simulink model "sampleModel2_EMI_Var"  (R2017a)
settings: Solver=VariableStepAuto  StartTime=0.0  StopTime=10.0  RelTol=1e-3
undefined symbols (not defined in the file or in its folder): DiscIntNeverNeededParam
libraries: simulink x42
settings Model: Creator=cyfuzz  LastModifiedBy=cyfuzz

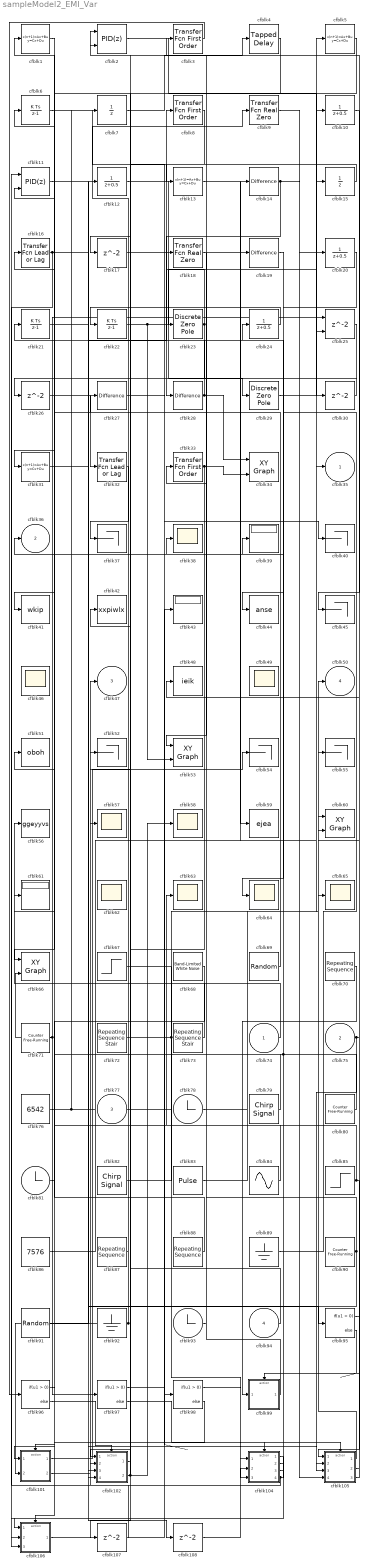
== system sampleModel2_EMI_Var ==
  cfblk74 : Inport
  cfblk75 : Inport  Port=2
  cfblk77 : Inport  Port=3
  cfblk94 : Inport  Port=4
  cfblk{1,5,13,31} (4 alike) : DiscreteStateSpace
  cfblk{10,12,20,24} (4 alike) : DiscreteTransferFcn  SampleTime=1
  cfblk101 : Subsystem  TreatAsAtomicUnit=on
  cfblk102 : Subsystem  TreatAsAtomicUnit=on
  cfblk104 : Subsystem  TreatAsAtomicUnit=on
  cfblk105 : Subsystem  TreatAsAtomicUnit=on
  cfblk106 : Subsystem  TreatAsAtomicUnit=on
  cfblk{17,26,30,107..108} (5 alike) : Delay  SampleTime=1
  cfblk11 : simulink/Continuous/PID Controller (2DOF)  Controller=PID  TimeDomain=Discrete-time  SampleTime=1  IntegratorMethod=Forward Euler  FilterMethod=Forward Euler  Form=Parallel  UseFilter=on  ControllerParametersSource=internal  P=1  I=1  D=0  N=100  b=1  c=1  InitialConditionSource=internal  InitialConditionForIntegrator=0  InitialConditionForFilter=0  ExternalReset=none  LimitOutput=off  UpperSaturationLimit=inf  LowerSaturationLimit=-inf  LinearizeAsGain=off  AntiWindupMode=none  Kb=1  TrackingMode=off  Kt=1  PParamMin=[]  PParamMax=[]  IParamMin=[]  IParamMax=[]  DParamMin=[]  DParamMax=[]  NParamMin=[]  NParamMax=[]  bParamMin=[]  bParamMax=[]  cParamMin=[]  cParamMax=[]  KbParamMin=[]  KbParamMax=[]  KtParamMin=[]  KtParamMax=[]  POutMin=[]  POutMax=[]  IOutMin=[]  IOutMax=[]  DOutMin=[]  DOutMax=[]  NOutMin=[]  NOutMax=[]  bOutMin=[]  bOutMax=[]  cOutMin=[]  cOutMax=[]  KbOutMin=[]  KbOutMax=[]  KtOutMin=[]  KtOutMax=[]  IntegratorOutMin=[]  IntegratorOutMax=[]  FilterOutMin=[]  FilterOutMax=[]  SumOutMin=[]  SumOutMax=[]  Sum1OutMin=[]  Sum1OutMax=[]  Sum2OutMin=[]  Sum2OutMax=[]  Sum3OutMin=[]  Sum3OutMax=[]  SumI1OutMin=[]  SumI1OutMax=[]  SumI2OutMin=[]  SumI2OutMax=[]  SumI3OutMin=[]  SumI3OutMax=[]  SumDOutMin=[]  SumDOutMax=[]  SaturationOutMin=[]  SaturationOutMax=[]  IntegratorContinuousStateAttributes=''  IntegratorStateMustResolveToSignalObject=off  IntegratorRTWStateStorageClass=Auto  FilterContinuousStateAttributes=''  FilterStateMustResolveToSignalObject=off  FilterRTWStateStorageClass=Auto  DifferentiatorICPrevScaledInput=0  DifferentiatorOutMin=[]  DifferentiatorOutMax=[]  InitialConditionSetting=State (most efficient)
  cfblk{14,19,27..28} (4 alike) : simulink/Discrete/Difference  ICPrevInput=0.0  OutMin=[]  OutMax=[]  OutDataTypeStr=Inherit: Inherit via back propagation  OutDataType=fixdt(1, 16)  OutScaling=2^-10  DoSatur=off
  cfblk15 : UnitDelay
  cfblk16 : simulink/Discrete/Transfer Fcn Lead or Lag  PoleZ=0.95  ZeroZ=0.75  ICPrevOutput=0.0  ICPrevInput=0.0  DoSatur=off
      settings: SourceProductName=Simulink  SourceProductBaseCode=SL
  cfblk18 : simulink/Discrete/Transfer Fcn Real Zero  ZeroZ=0.75  ICPrevInput=0.0  DoSatur=off
      settings: SourceProductName=Simulink  SourceProductBaseCode=SL
  cfblk2 : simulink/Continuous/PID Controller (2DOF)  Controller=PID  TimeDomain=Discrete-time  SampleTime=1  IntegratorMethod=Forward Euler  FilterMethod=Forward Euler  Form=Parallel  UseFilter=on  ControllerParametersSource=internal  P=1  I=1  D=0  N=100  b=1  c=1  InitialConditionSource=internal  InitialConditionForIntegrator=0  InitialConditionForFilter=0  ExternalReset=none  LimitOutput=off  UpperSaturationLimit=inf  LowerSaturationLimit=-inf  LinearizeAsGain=off  AntiWindupMode=none  Kb=1  TrackingMode=off  Kt=1  PParamMin=[]  PParamMax=[]  IParamMin=[]  IParamMax=[]  DParamMin=[]  DParamMax=[]  NParamMin=[]  NParamMax=[]  bParamMin=[]  bParamMax=[]  cParamMin=[]  cParamMax=[]  KbParamMin=[]  KbParamMax=[]  KtParamMin=[]  KtParamMax=[]  POutMin=[]  POutMax=[]  IOutMin=[]  IOutMax=[]  DOutMin=[]  DOutMax=[]  NOutMin=[]  NOutMax=[]  bOutMin=[]  bOutMax=[]  cOutMin=[]  cOutMax=[]  KbOutMin=[]  KbOutMax=[]  KtOutMin=[]  KtOutMax=[]  IntegratorOutMin=[]  IntegratorOutMax=[]  FilterOutMin=[]  FilterOutMax=[]  SumOutMin=[]  SumOutMax=[]  Sum1OutMin=[]  Sum1OutMax=[]  Sum2OutMin=[]  Sum2OutMax=[]  Sum3OutMin=[]  Sum3OutMax=[]  SumI1OutMin=[]  SumI1OutMax=[]  SumI2OutMin=[]  SumI2OutMax=[]  SumI3OutMin=[]  SumI3OutMax=[]  SumDOutMin=[]  SumDOutMax=[]  SaturationOutMin=[]  SaturationOutMax=[]  IntegratorContinuousStateAttributes=''  IntegratorStateMustResolveToSignalObject=off  IntegratorRTWStateStorageClass=Auto  FilterContinuousStateAttributes=''  FilterStateMustResolveToSignalObject=off  FilterRTWStateStorageClass=Auto  DifferentiatorICPrevScaledInput=0  DifferentiatorOutMin=[]  DifferentiatorOutMax=[]  InitialConditionSetting=State (most efficient)
  cfblk21 : DiscreteIntegrator  InitialConditionSetting=State (most efficient)  ICPrevOutput=DiscIntNeverNeededParam  ICPrevScaledInput=DiscIntNeverNeededParam
  cfblk22 : DiscreteIntegrator  InitialConditionSetting=State (most efficient)  ICPrevOutput=DiscIntNeverNeededParam  ICPrevScaledInput=DiscIntNeverNeededParam
  cfblk23 : DiscreteZeroPole  Poles=[0 0.5]  Gain=1
  cfblk25 : Delay  ShowEnablePort=on  SampleTime=1
      settings: InputPortMap=u0,e6
  cfblk29 : DiscreteZeroPole  Poles=[0 0.5]  Gain=1
  cfblk3 : simulink/Discrete/Transfer Fcn First Order  PoleZ=0.95  ICPrevOutput=0.0  DoSatur=off
      settings: SourceProductName=Simulink
  cfblk32 : simulink/Discrete/Transfer Fcn Lead or Lag  PoleZ=0.95  ZeroZ=0.75  ICPrevOutput=0.0  ICPrevInput=0.0  DoSatur=off
      settings: SourceProductName=Simulink  SourceProductBaseCode=SL
  cfblk33 : simulink/Discrete/Transfer Fcn First Order  PoleZ=0.95  ICPrevOutput=0.0  DoSatur=off
      settings: SourceProductName=Simulink
  cfblk{34,53,60,66} (4 alike) : simulink/Sinks/XY Graph  xmin=-1  xmax=1  ymin=-1  ymax=1  st=-1
  cfblk{37,40,45,52,54..55} (6 alike) : Terminator
  cfblk{38,46,49,57..58,62..65} (9 alike) : Scope
      cfblk46 settings: Floating=on
      cfblk49 settings: Floating=on
      cfblk62 settings: Floating=on
  cfblk39 : Display
  cfblk4 : simulink/Discrete/Tapped Delay  vinit=0.0  samptime=-1  NumDelays=1  DelayOrder=Oldest  includeCurrent=off
  cfblk41 : ToFile  Filename=wkip  SaveFormat=Timeseries
  cfblk42 : ToWorkspace  VariableName=xxpiwlx  SaveFormat=Timeseries  SampleTime=-1
  cfblk43 : Display
  cfblk44 : ToFile  Filename=anse  SaveFormat=Timeseries
  cfblk48 : ToFile  Filename=ieik  SaveFormat=Timeseries
  cfblk51 : ToFile  Filename=oboh  SaveFormat=Timeseries
  cfblk56 : ToWorkspace  VariableName=ggeyyvs  SaveFormat=Timeseries  SampleTime=-1
  cfblk59 : ToFile  Filename=ejea  SaveFormat=Timeseries
  cfblk6 : DiscreteIntegrator  InitialConditionSetting=State (most efficient)  ICPrevOutput=DiscIntNeverNeededParam  ICPrevScaledInput=DiscIntNeverNeededParam
  cfblk61 : Display
  cfblk67 : Step  After=37  SampleTime=0
  cfblk68 : simulink/Sources/Band-Limited White Noise  Cov=[0.1]  Ts=0.1  seed=[23341]
  cfblk69 : UniformRandomNumber  SampleTime=0.1
  cfblk7 : UnitDelay
  cfblk70 : simulink/Sources/Repeating Sequence  rep_seq_t=[0 2]  rep_seq_y=[0 2]
  cfblk71 : simulink/Sources/Counter Free-Running  NumBits=16  tsamp=-1
  cfblk72 : simulink/Sources/Repeating Sequence Stair  OutValues=[3 1 4 2 1].'  tsamp=-1  OutMin=[]  OutMax=[]  OutDataTypeStr=double  OutputDataTypeScalingMode=double  OutDataType=fixdt(0,8)  ConRadixGroup=Best Precision: Vector-wise  OutScaling=2^-12
  cfblk73 : simulink/Sources/Repeating Sequence Stair  OutValues=[3 1 4 2 1].'  tsamp=-1  OutMin=[]  OutMax=[]  OutDataTypeStr=double  OutputDataTypeScalingMode=double  OutDataType=fixdt(0,8)  ConRadixGroup=Best Precision: Vector-wise  OutScaling=2^-12
  cfblk76 : Constant  Value=6542
  cfblk78 : Clock
  cfblk79 : simulink/Sources/Chirp Signal  f1=0.1  T=100  f2=1
  cfblk8 : simulink/Discrete/Transfer Fcn First Order  PoleZ=0.95  ICPrevOutput=0.0  DoSatur=off
      settings: SourceProductName=Simulink
  cfblk80 : simulink/Sources/Counter Free-Running  NumBits=16  tsamp=-1
  cfblk81 : Clock
  cfblk82 : simulink/Sources/Chirp Signal  f1=0.1  T=100  f2=1
  cfblk83 : DiscretePulseGenerator  PulseType=Time based  Period=10  PulseWidth=5
  cfblk84 : Sin  SampleTime=0
  cfblk85 : Step  After=57  SampleTime=0
  cfblk86 : Constant  Value=7576
  cfblk87 : simulink/Sources/Repeating Sequence  rep_seq_t=[0 2]  rep_seq_y=[0 2]
  cfblk88 : simulink/Sources/Repeating Sequence  rep_seq_t=[0 2]  rep_seq_y=[0 2]
  cfblk89 : Ground
  cfblk9 : simulink/Discrete/Transfer Fcn Real Zero  ZeroZ=0.75  ICPrevInput=0.0  DoSatur=off
      settings: SourceProductName=Simulink  SourceProductBaseCode=SL
  cfblk90 : simulink/Sources/Counter Free-Running  NumBits=16  tsamp=-1
  cfblk91 : RandomNumber  SampleTime=0.1
  cfblk92 : Ground
  cfblk93 : Clock
  cfblk{95..98} (4 alike) : If  SampleTime=1
  cfblk99 : Subsystem  TreatAsAtomicUnit=on
  cfblk35 : Outport
  cfblk36 : Outport  Port=2
  cfblk47 : Outport  Port=3
  cfblk50 : Outport  Port=4
  wires:
  cfblk73/1 -> cfblk56/1
  cfblk99/1(cfblk2) -> cfblk33/1
  cfblk12/1 -> cfblk29/1
  cfblk77/1 -> cfblk50/1
  cfblk89/1 -> cfblk24/1
  cfblk104/1(cfblk2) -> cfblk106/1(cfblk1)
  cfblk17/1 -> cfblk9/1
  cfblk75/1 -> cfblk2/1, cfblk105/3(cfblk8)
  cfblk28/1 -> cfblk8/1, cfblk34/1
  cfblk70/1 -> cfblk99/1(cfblk1)
  cfblk14/1 -> cfblk28/1, cfblk105/4(cfblk9)
  cfblk104/2(cfblk9) -> cfblk36/1
  cfblk33/1 -> cfblk34/2, cfblk107/1
  cfblk3/1 -> cfblk96/1
  cfblk105/1(cfblk2) -> cfblk55/1
  cfblk9/1 -> cfblk20/1
  cfblk101/1(cfblk2) -> cfblk54/1
  cfblk101/2(cfblk7) -> cfblk47/1
  cfblk86/1 -> cfblk14/1
  cfblk30/1 -> cfblk26/1
  cfblk91/1 -> cfblk12/1
  cfblk84/1 -> cfblk51/1
  cfblk5/1 -> cfblk66/1
  cfblk67/1 -> cfblk104/1(cfblk1)
  cfblk85/1 -> cfblk63/1, cfblk105/1(cfblk1)
  cfblk11/1 -> cfblk95/1
  cfblk78/1 -> cfblk35/1
  cfblk94/1 -> cfblk42/1
  cfblk102/1(cfblk2) -> cfblk2/2
  cfblk2/1 -> cfblk30/1
  cfblk13/1 -> cfblk59/1
  cfblk76/1 -> cfblk10/1, cfblk7/1
  cfblk23/1 -> cfblk18/1, cfblk102/3(cfblk12)
  cfblk26/1 -> cfblk32/1
  cfblk79/1 -> cfblk27/1
  cfblk15/1 -> cfblk13/1
  cfblk22/1 -> cfblk5/1, cfblk53/2
  cfblk19/1 -> cfblk64/1
  cfblk83/1 -> cfblk60/1
  cfblk24/1 -> cfblk22/1
  cfblk25/1 -> cfblk41/1
  cfblk20/1 -> cfblk44/1
  cfblk18/1 -> cfblk53/1
  cfblk32/1 -> cfblk37/1
  cfblk106/1(cfblk2) -> cfblk43/1
  cfblk105/2(cfblk10) -> cfblk60/2
  cfblk74/1 -> cfblk16/1
  cfblk90/1 -> cfblk3/1, cfblk102/4(cfblk13)
  cfblk102/2(cfblk14) -> cfblk52/1, cfblk58/1
  cfblk104/3(cfblk10) -> cfblk106/2(cfblk7)
  cfblk1/1 -> cfblk31/1
  cfblk10/1 -> cfblk45/1
  cfblk29/1 -> cfblk15/1
  cfblk88/1 -> cfblk6/1
  cfblk72/1 -> cfblk65/1, cfblk105/2(cfblk7)
  cfblk105/3(cfblk11) -> cfblk48/1
  cfblk27/1 -> cfblk40/1
  cfblk87/1 -> cfblk57/1
  cfblk6/1 -> cfblk98/1
  cfblk4/1 -> cfblk102/1(cfblk1)
  cfblk82/1 -> cfblk25/2
  cfblk68/1 -> cfblk101/1(cfblk1)
  cfblk8/1 -> cfblk17/1
  cfblk69/1 -> cfblk11/2
  cfblk104/4(cfblk11) -> cfblk21/1, cfblk102/2(cfblk11)
  cfblk81/1 -> cfblk1/1
  cfblk31/1 -> cfblk23/1
  cfblk16/1 -> cfblk106/3(cfblk8), cfblk104/3(cfblk8)
  cfblk7/1 -> cfblk4/1
  cfblk80/1 -> cfblk39/1, cfblk61/1
  cfblk93/1 -> cfblk38/1
  cfblk95/1 -> cfblk99/Action
  cfblk95/2 -> ?
  cfblk96/1 -> cfblk101/Action
  cfblk96/2 -> cfblk102/Action
  cfblk97/1 -> ?
  cfblk97/2 -> cfblk104/Action
  cfblk98/1 -> cfblk105/Action
  cfblk98/2 -> cfblk106/Action
  cfblk107/1 -> cfblk11/1
  cfblk21/1 -> cfblk108/1
  cfblk108/1 -> cfblk104/2(cfblk7)
  cfblk71/1 -> cfblk66/2, cfblk97/1, cfblk25/1
  cfblk92/1 -> cfblk101/2(cfblk6), cfblk19/1

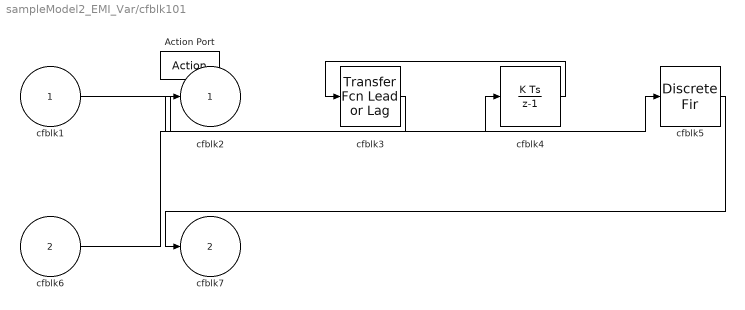
== system sampleModel2_EMI_Var/cfblk101 ==
  cfblk1 : Inport
  cfblk6 : Inport  Port=2
  Action Port : ActionPort  ActionType=then
  cfblk3 : simulink/Discrete/Transfer Fcn Lead or Lag  PoleZ=0.95  ZeroZ=0.75  ICPrevOutput=0.0  ICPrevInput=0.0  DoSatur=off
      settings: SourceProductName=Simulink  SourceProductBaseCode=SL
  cfblk4 : DiscreteIntegrator  InitialConditionSetting=State (most efficient)  SampleTime=-1  ICPrevOutput=DiscIntNeverNeededParam  ICPrevScaledInput=DiscIntNeverNeededParam
  cfblk5 : DiscreteFir
  cfblk2 : Outport
  cfblk7 : Outport  Port=2
  wires:
  cfblk1/1 -> cfblk5/1
  cfblk5/1 -> cfblk7/1
  cfblk4/1 -> cfblk3/1
  cfblk3/1 -> cfblk2/1
  cfblk6/1 -> cfblk4/1

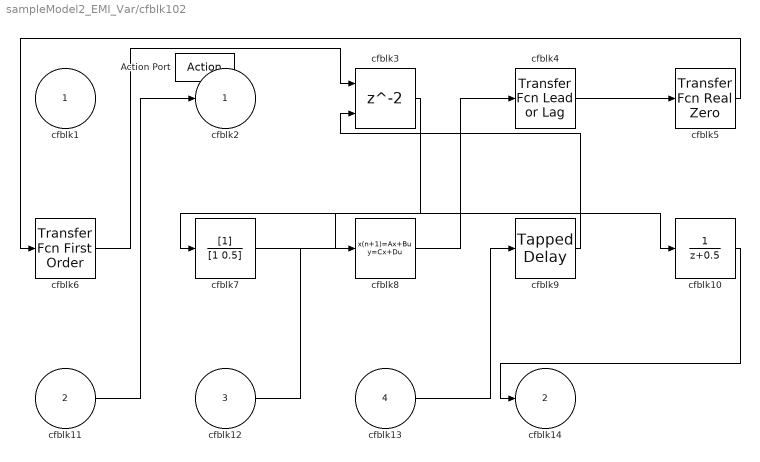
== system sampleModel2_EMI_Var/cfblk102 ==
  cfblk1 : Inport
  cfblk11 : Inport  Port=2
  cfblk12 : Inport  Port=3
  cfblk13 : Inport  Port=4
  Action Port : ActionPort  ActionType=else
  cfblk10 : DiscreteTransferFcn
  cfblk3 : Delay  ShowEnablePort=on
      settings: InputPortMap=u0,e6
  cfblk4 : simulink/Discrete/Transfer Fcn Lead or Lag  PoleZ=0.95  ZeroZ=0.75  ICPrevOutput=0.0  ICPrevInput=0.0  DoSatur=off
      settings: SourceProductName=Simulink  SourceProductBaseCode=SL
  cfblk5 : simulink/Discrete/Transfer Fcn Real Zero  ZeroZ=0.75  ICPrevInput=0.0  DoSatur=off
      settings: SourceProductName=Simulink  SourceProductBaseCode=SL
  cfblk6 : simulink/Discrete/Transfer Fcn First Order  PoleZ=0.95  ICPrevOutput=0.0  DoSatur=off
      settings: SourceProductName=Simulink
  cfblk7 : DiscreteFilter
  cfblk8 : DiscreteStateSpace  SampleTime=-1
  cfblk9 : simulink/Discrete/Tapped Delay  vinit=0.0  samptime=-1  NumDelays=1  DelayOrder=Oldest  includeCurrent=off
  cfblk2 : Outport
  cfblk14 : Outport  Port=2
  wires:
  cfblk8/1 -> cfblk4/1
  cfblk10/1 -> cfblk14/1
  cfblk4/1 -> cfblk5/1
  cfblk13/1 -> cfblk9/1
  cfblk3/1 -> cfblk7/1
  cfblk11/1 -> cfblk2/1
  cfblk12/1 -> cfblk8/1
  cfblk6/1 -> cfblk3/1
  cfblk9/1 -> cfblk3/2
  cfblk5/1 -> cfblk6/1
  cfblk7/1 -> cfblk10/1

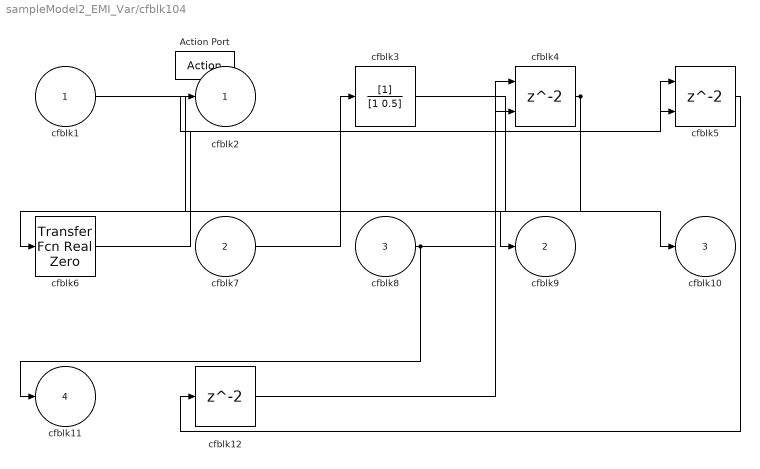
== system sampleModel2_EMI_Var/cfblk104 ==
  cfblk1 : Inport
  cfblk7 : Inport  Port=2
  cfblk8 : Inport  Port=3
  Action Port : ActionPort  ActionType=else
  cfblk12 : Delay
  cfblk3 : DiscreteFilter
  cfblk4 : Delay  ShowEnablePort=on
      settings: InputPortMap=u0,e6
  cfblk5 : Delay  ShowEnablePort=on
      settings: InputPortMap=u0,e6
  cfblk6 : simulink/Discrete/Transfer Fcn Real Zero  ZeroZ=0.75  ICPrevInput=0.0  DoSatur=off
      settings: SourceProductName=Simulink  SourceProductBaseCode=SL
  cfblk2 : Outport
  cfblk9 : Outport  Port=2
  cfblk10 : Outport  Port=3
  cfblk11 : Outport  Port=4
  wires:
  cfblk6/1 -> cfblk5/1
  cfblk1/1 -> cfblk9/1
  cfblk3/1 -> cfblk10/1
  cfblk8/1 -> cfblk4/2, cfblk5/2, cfblk11/1
  cfblk4/1 -> cfblk2/1, cfblk6/1
  cfblk7/1 -> cfblk3/1
  cfblk5/1 -> cfblk12/1
  cfblk12/1 -> cfblk4/1

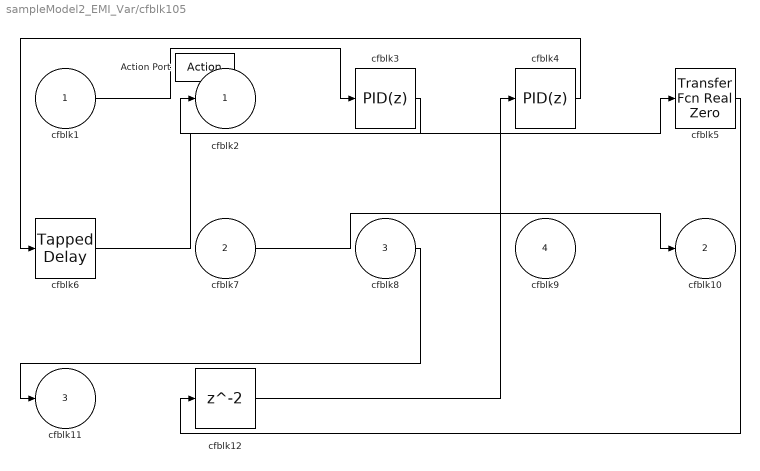
== system sampleModel2_EMI_Var/cfblk105 ==
  cfblk1 : Inport
  cfblk7 : Inport  Port=2
  cfblk8 : Inport  Port=3
  cfblk9 : Inport  Port=4
  Action Port : ActionPort  ActionType=then
  cfblk12 : Delay
  cfblk3 : simulink/Continuous/PID Controller  Controller=PID  TimeDomain=Discrete-time  SampleTime=-1  IntegratorMethod=Forward Euler  FilterMethod=Forward Euler  Form=Parallel  UseFilter=on  ControllerParametersSource=internal  P=1  I=1  D=0  N=100  InitialConditionSource=internal  InitialConditionForIntegrator=0  InitialConditionForFilter=0  ExternalReset=none  LimitOutput=off  UpperSaturationLimit=inf  LowerSaturationLimit=-inf  LinearizeAsGain=off  AntiWindupMode=none  Kb=1  TrackingMode=off  Kt=1  PParamMin=[]  PParamMax=[]  IParamMin=[]  IParamMax=[]  DParamMin=[]  DParamMax=[]  NParamMin=[]  NParamMax=[]  KbParamMin=[]  KbParamMax=[]  KtParamMin=[]  KtParamMax=[]  POutMin=[]  POutMax=[]  IOutMin=[]  IOutMax=[]  DOutMin=[]  DOutMax=[]  NOutMin=[]  NOutMax=[]  KbOutMin=[]  KbOutMax=[]  KtOutMin=[]  KtOutMax=[]  IntegratorOutMin=[]  IntegratorOutMax=[]  FilterOutMin=[]  FilterOutMax=[]  SumOutMin=[]  SumOutMax=[]  SumI1OutMin=[]  SumI1OutMax=[]  SumI2OutMin=[]  SumI2OutMax=[]  SumI3OutMin=[]  SumI3OutMax=[]  SumDOutMin=[]  SumDOutMax=[]  SaturationOutMin=[]  SaturationOutMax=[]  IntegratorContinuousStateAttributes=''  IntegratorStateMustResolveToSignalObject=off  IntegratorRTWStateStorageClass=Auto  FilterContinuousStateAttributes=''  FilterStateMustResolveToSignalObject=off  FilterRTWStateStorageClass=Auto  DifferentiatorICPrevScaledInput=0  DifferentiatorOutMin=[]  DifferentiatorOutMax=[]  InitialConditionSetting=State (most efficient)
  cfblk4 : simulink/Continuous/PID Controller  Controller=PID  TimeDomain=Discrete-time  SampleTime=-1  IntegratorMethod=Forward Euler  FilterMethod=Forward Euler  Form=Parallel  UseFilter=on  ControllerParametersSource=internal  P=1  I=1  D=0  N=100  InitialConditionSource=internal  InitialConditionForIntegrator=0  InitialConditionForFilter=0  ExternalReset=none  LimitOutput=off  UpperSaturationLimit=inf  LowerSaturationLimit=-inf  LinearizeAsGain=off  AntiWindupMode=none  Kb=1  TrackingMode=off  Kt=1  PParamMin=[]  PParamMax=[]  IParamMin=[]  IParamMax=[]  DParamMin=[]  DParamMax=[]  NParamMin=[]  NParamMax=[]  KbParamMin=[]  KbParamMax=[]  KtParamMin=[]  KtParamMax=[]  POutMin=[]  POutMax=[]  IOutMin=[]  IOutMax=[]  DOutMin=[]  DOutMax=[]  NOutMin=[]  NOutMax=[]  KbOutMin=[]  KbOutMax=[]  KtOutMin=[]  KtOutMax=[]  IntegratorOutMin=[]  IntegratorOutMax=[]  FilterOutMin=[]  FilterOutMax=[]  SumOutMin=[]  SumOutMax=[]  SumI1OutMin=[]  SumI1OutMax=[]  SumI2OutMin=[]  SumI2OutMax=[]  SumI3OutMin=[]  SumI3OutMax=[]  SumDOutMin=[]  SumDOutMax=[]  SaturationOutMin=[]  SaturationOutMax=[]  IntegratorContinuousStateAttributes=''  IntegratorStateMustResolveToSignalObject=off  IntegratorRTWStateStorageClass=Auto  FilterContinuousStateAttributes=''  FilterStateMustResolveToSignalObject=off  FilterRTWStateStorageClass=Auto  DifferentiatorICPrevScaledInput=0  DifferentiatorOutMin=[]  DifferentiatorOutMax=[]  InitialConditionSetting=State (most efficient)
  cfblk5 : simulink/Discrete/Transfer Fcn Real Zero  ZeroZ=0.75  ICPrevInput=0.0  DoSatur=off
      settings: SourceProductName=Simulink  SourceProductBaseCode=SL
  cfblk6 : simulink/Discrete/Tapped Delay  vinit=0.0  samptime=-1  NumDelays=1  DelayOrder=Oldest  includeCurrent=off
  cfblk2 : Outport
  cfblk10 : Outport  Port=2
  cfblk11 : Outport  Port=3
  wires:
  cfblk6/1 -> cfblk5/1
  cfblk1/1 -> cfblk3/1
  cfblk3/1 -> cfblk2/1
  cfblk4/1 -> cfblk6/1
  cfblk8/1 -> cfblk11/1
  cfblk7/1 -> cfblk10/1
  cfblk5/1 -> cfblk12/1
  cfblk12/1 -> cfblk4/1

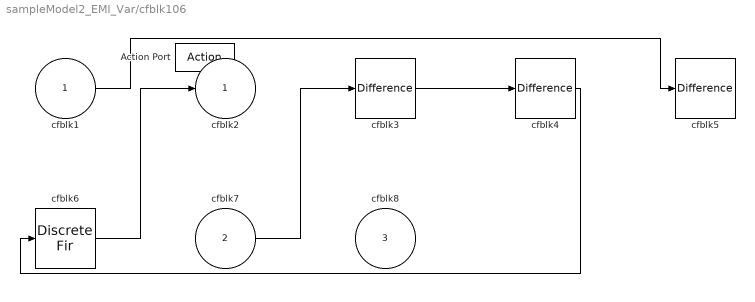
== system sampleModel2_EMI_Var/cfblk106 ==
  cfblk1 : Inport
  cfblk7 : Inport  Port=2
  cfblk8 : Inport  Port=3
  Action Port : ActionPort  ActionType=else
  cfblk3 : simulink/Discrete/Difference  ICPrevInput=0.0  OutMin=[]  OutMax=[]  OutDataTypeStr=Inherit: Inherit via back propagation  OutDataType=fixdt(1, 16)  OutScaling=2^-10  DoSatur=off
  cfblk4 : simulink/Discrete/Difference  ICPrevInput=0.0  OutMin=[]  OutMax=[]  OutDataTypeStr=Inherit: Inherit via back propagation  OutDataType=fixdt(1, 16)  OutScaling=2^-10  DoSatur=off
  cfblk5 : simulink/Discrete/Difference  ICPrevInput=0.0  OutMin=[]  OutMax=[]  OutDataTypeStr=Inherit: Inherit via back propagation  OutDataType=fixdt(1, 16)  OutScaling=2^-10  DoSatur=off
  cfblk6 : DiscreteFir
  cfblk2 : Outport
  wires:
  cfblk3/1 -> cfblk4/1
  cfblk6/1 -> cfblk2/1
  cfblk4/1 -> cfblk6/1
  cfblk7/1 -> cfblk3/1
  cfblk1/1 -> cfblk5/1

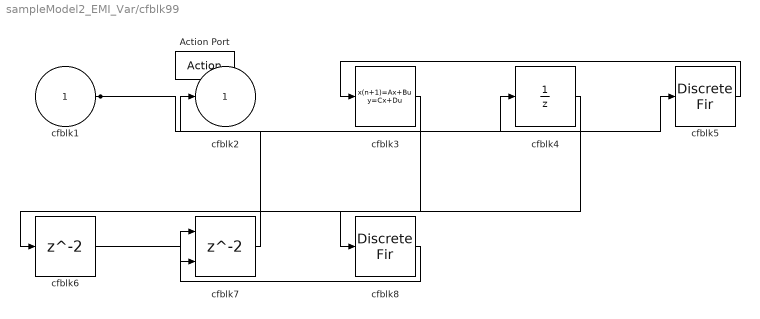
== system sampleModel2_EMI_Var/cfblk99 ==
  cfblk1 : Inport
  Action Port : ActionPort  ActionType=then
  cfblk3 : DiscreteStateSpace  SampleTime=-1
  cfblk4 : UnitDelay  SampleTime=-1
  cfblk5 : DiscreteFir
  cfblk6 : Delay
  cfblk7 : Delay  ShowEnablePort=on
      settings: InputPortMap=u0,e6
  cfblk8 : DiscreteFir
  cfblk2 : Outport
  wires:
  cfblk4/1 -> cfblk8/1
  cfblk7/1 -> cfblk2/1
  cfblk8/1 -> cfblk7/1
  cfblk5/1 -> cfblk3/1
  cfblk3/1 -> cfblk6/1
  cfblk6/1 -> cfblk7/2
  cfblk1/1 -> cfblk5/1, cfblk4/1
